simulink model "atrias_system_4khz"  (R2016b)
settings: Solver=FixedStepDiscrete  StartTime=0.0  StopTime=inf  FixedStep=elmo_sample_time  RelTol=1e-3
undefined symbols (not defined in the file or in its folder): gui_disable_cmd, gui_enable_cmd, gui_exit_cmd, gui_reset_cmd, HARD_MOTOR_POSITION_LIMITS_LOWER, HARD_MOTOR_POSITION_LIMITS_UPPER, HIP_ABS_MAX_ENCODER_TICKS, HIP_CURRENT_LIMIT, HIP_INC_MAX_ENCODER_TICKS, HIP_MOTOR_CONSTANT, HIP_MTR_GEAR_RATIO, HIP_MTR_MAX_TORQUE, LEFT_MOTOR_HIP_DIRECTION, LEG1_MOTOR_A_DIRECTION, LEG1_MOTOR_B_DIRECTION, LEG2_MOTOR_A_DIRECTION, LEG2_MOTOR_B_DIRECTION, LEG_CURRENT_LIMIT, LEG_INC_ENCODER_DIRECTION_LEFT_BACK, LEG_INC_ENCODER_DIRECTION_LEFT_FRONT, LEG_INC_ENCODER_DIRECTION_RIGHT_BACK, LEG_INC_ENCODER_DIRECTION_RIGHT_FRONT, LEG_INC_ENCODER_RAD_PER_TICK, LEG_MOTOR_CONSTANT, LEG_MTR_GEAR_RATIO, LEG_MTR_MAX_TORQUE, max_hip_velocity, max_motor_velocity, MEDULLA_ADC_MAX_VOLTS, MEDULLA_ADC_OFFSET_COUNTS, MEDULLA_STATE_ERROR, MEDULLA_STATE_HALT, MEDULLA_STATE_IDLE, MEDULLA_STATE_RESET, MEDULLA_STATE_RUN, MOTOR_POSITION_LIMITS_LOWER, MOTOR_POSITION_LIMITS_UPPER, MTR_HIP_MAX_CURRENT, MTR_MAX_CONT_CURRENT, MTR_MAX_COUNT, MTR_MAX_CURRENT, MTR_MAX_TEMP, RIGHT_MOTOR_HIP_DIRECTION
libraries: xpcethercatlib x190, simulink x37
(part 4 of 4)

== matlab function atrias_system_4khz/Demux Diags ==
  data: diags input; halt_diag output; sw1 output; sw2 output; sw3 output; sw4 output; error1 output; error2 output; error3 output; error4 output; error5 output; error6 output; error7 output; contrlr_fault_diag output; softLimits output; decelFailEstop output; transmissionLimits output
function [halt_diag,sw1,sw2,sw3,sw4,error1,error2,error3,error4,error5,error6,error7,contrlr_fault_diag,softLimits,decelFailEstop,transmissionLimits] = fcn(diags)
%#codegen

halt_diag          = diags(1);
sw1                = diags(2:9);
sw2                = diags(10:17);
sw3                = diags(18:25);
sw4                = diags(26:33);
error1             = diags(34:41);
error2             = diags(42:49);
error3             = diags(50:57);
error4             = diags(58:65);
error5             = diags(66:73);
error6             = diags(74:81);
error7             = diags(82:89);
contrlr_fault_diag = diags(90);
softLimits         = diags(91:102);
decelFailEstop     = diags(103);
transmissionLimits = diags(104:111);

== matlab function atrias_system_4khz/DAQ/battery_ADC_to_volts ==
  data: u input; volt output
function volt = fcn(u)
% Linear fit determined experimentally
volt = (u-445)*0.0266; % [V]

== matlab function atrias_system_4khz/DAQ/battery_ADC_to_current ==
  data: u input; amps output
function amps = fcn(u)
% Linear fit determined experimentally
amps = (u-2015)*(2.29/20); % [V]

== matlab function atrias_system_4khz/Soft Limits ==
  data: estop output; q input; rotorPos input; rotorVel input; runCommand input; halt output; MOTOR_POSITION_LIMITS_UPPER parameter double; MOTOR_POSITION_LIMITS_LOWER parameter double; motorLimits output; transmissionLimits output
function [estop,halt,motorLimits,transmissionLimits] = fcn(q, ...
                                  rotorPos, ...
                                  rotorVel, ...
                                  runCommand, ...
                                  MOTOR_POSITION_LIMITS_UPPER, ...
                                  MOTOR_POSITION_LIMITS_LOWER)


%% Check the deflection between the incremental and absolute positions
% q: rBl rBm rAl rAm lBl lBm lAl lAm rHm lHm bR bY bP
% rotor: rBr rAr lBr lAr rHr lHr
% Sanity check absolute angles w.r.t. incremental angles
transmissionDfl = rotorPos(1:4) - q([2 4 6 8]);

transmissionLimits = [transmissionDfl > 0.1
                      transmissionDfl < -0.1];

% Estop if any sensors are reporting weird data
estop = any(transmissionLimits);

% Handle encoder spikes
persistent count;
if isempty(count); count = 0; end
% If in run
if runCommand == true
    % If estop is thrown and there haven't been many bad cycles
    if estop && (count < 10)
        % Ignore the transmission limits
        estop = false;
        transmissionLimits = transmissionLimits & false;
        % Increment the count
        count = count + 1;
    end
    % If count is non-zero but estop has not been thrown
    if ~estop && (count ~= 0)
        % Reset the count
        count = 0;
    end
else % If not in run
    % Reset the counter
    count = 0;
end % if runCommand

%% Predicted stopping location at max deceleration [rad]
%    Current position + average velocity * speed   / deceleration rate
%    [rad]            + [rad/s]          * [rad/s] / ([rad/s^2/A] * [A])
rb = rotorPos(1) + rotorVel(1)/2 * abs(rotorVel(1)) / (1.7185879 * 100.0);
ra = rotorPos(2) + rotorVel(2)/2 * abs(rotorVel(2)) / (1.7185879 * 100.0);
lb = rotorPos(3) + rotorVel(3)/2 * abs(rotorVel(3)) / (1.7185879 * 100.0);
la = rotorPos(4) + rotorVel(4)/2 * abs(rotorVel(4)) / (1.7185879 * 100.0);

% Leg extension/retraction
rd = rb - ra;
ld = lb - la;

r = [ra; rb; rd];
l = [la; lb; ld];

% Check if any predicted angles are outside the safety limits
motorLimits = [r > MOTOR_POSITION_LIMITS_UPPER
               r < MOTOR_POSITION_LIMITS_LOWER
               l > MOTOR_POSITION_LIMITS_UPPER
               l < MOTOR_POSITION_LIMITS_LOWER];

halt = any(motorLimits);

end % function fcn

== matlab function atrias_system_4khz/Active Damping Safety ==
  data: tau input; tau_out output; rotorDQ input; isHalting input; decelFailEstop output
function [tau_out,decelFailEstop] = fcn(tau,rotorDQ,isHalting)

% rotor: rBr rAr lBr lAr rHr lHr
% torque: rB rA rH lB lA lH

% Deceleration initialization
persistent rB rA lB lA;
if isempty(rB)
    % Set the minimum allowable rotor velocity
    vMin = 0.3;
    rB = DampingCheck(vMin);
    rA = DampingCheck(vMin);
    lB = DampingCheck(vMin);
    lA = DampingCheck(vMin);
    % Set the current velocity as the initial velocity
    rB.initialVelocity(rotorDQ(1));
    rA.initialVelocity(rotorDQ(2));
    lB.initialVelocity(rotorDQ(3));
    lA.initialVelocity(rotorDQ(4));
end

% If everything is fine, act as a passthrough
if isHalting == false
    tau_out = tau;
    decelFailEstop = false;
    % Set the current velocity as the initial velocity
    rB.initialVelocity(rotorDQ(1));
    rA.initialVelocity(rotorDQ(2));
    lB.initialVelocity(rotorDQ(3));
    lA.initialVelocity(rotorDQ(4));
    return
end

% Damp if halting
kdlr = 600; % kd leg rotor
kdhr = 50;  % kd hip rotor
tau_out = (0 - rotorDQ([1 2 5 3 4 6])).*[kdlr kdlr kdhr kdlr kdlr kdhr]';

% E-stop if the robot fails to decelerate
decelFailTemp = [rB.checkDeceleration(rotorDQ(1))
                  rA.checkDeceleration(rotorDQ(2))
                  lB.checkDeceleration(rotorDQ(3))
                  lA.checkDeceleration(rotorDQ(4))];
decelFailEstop = any(decelFailTemp);
end % fcn
